simulink model "GEO_insertion"  (R2023b)
settings: Solver=FixedStepAuto  StartTime=0.0  StopTime=60*60*24*20  FixedStep=60  RelTol=1e-3
values from neighbouring files (symbols this model uses):
  A = 42164500    [GEO_insertion_setup.m]
  ext_ENV_muEarth = 3.986005e14    (= 398600500000000)    [GEO_insertion_setup.m]    (also in HSat_op_setup.m; HSat_op_setup_merged_maria.m; init_orbit_analysis_with_drag_loss.m)
  lambda_GEO = 79*pi/180    (= 1.37881010908)    [GEO_insertion_setup.m]
  OR_thrusterforce = 50e-3    (= 0.05)    [GEO_insertion_setup.m]    (also in HSat_op_setup.m = 0.275; HSat_op_setup_merged_maria.m = 0.275)
  psi_rads = 7.2921e-05    [GEO_insertion_setup.m]
  SC_mass = 500    [GEO_insertion_setup.m]
  sim_start = juliandate(2020, 1, 1, 12, 0, 0)    [GEO_insertion_setup.m]    (also in HSat_op_setup.m = ymd2jd(YYYY,MM,DD,'gregorian')-.5+hh/24+mm/1440+ss/86400; HSat_op_setup_merged_maria.m = ymd2jd(YYYY,MM,DD,'gregorian')-.5+hh/24+mm/1440+ss/86400)
  thrust_acc = OR_thrusterforce/SC_mass    (= 0.0001)    [GEO_insertion_setup.m]
undefined symbols (not defined in the file or in its folder): pos_start, vel_start
libraries: simulink x4, aerolibutil x2, sharedtransform x1, matrix_library x1
(part 1 of 2)
settings Model: Creator=mariahoflund  LastModifiedBy=mariahoflund

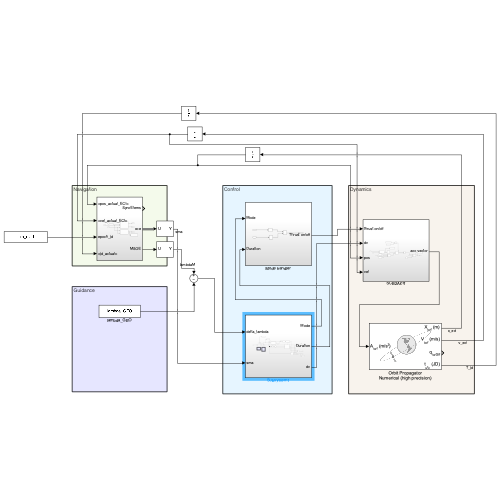
[thumbnail: Simulink's stored preview of the top-level diagram]
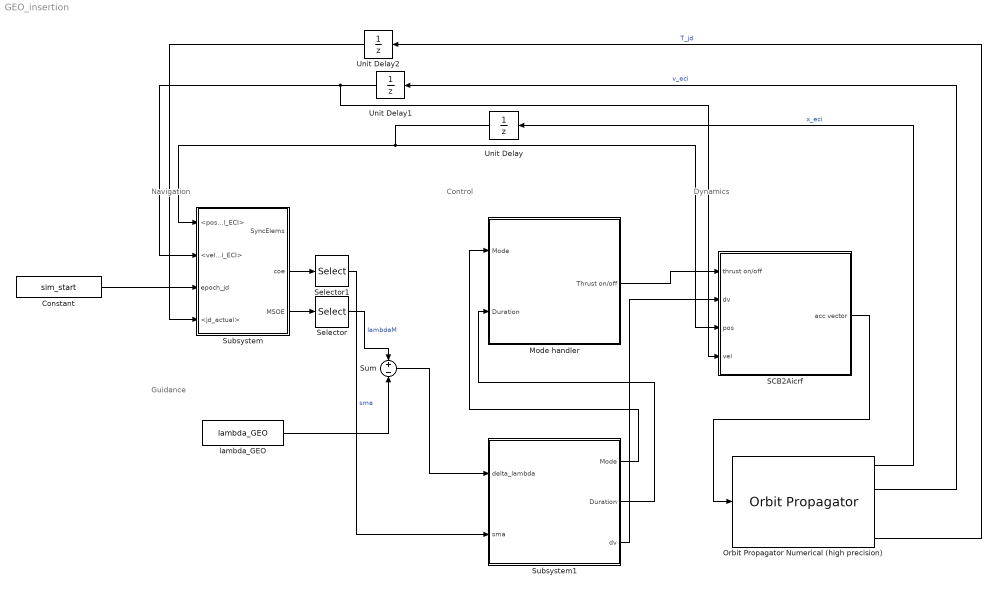
== system GEO_insertion ==
  note: Dynamics
  note: Control
  note: Navigation
  note: Guidance
  Constant : Constant  Value=sim_start
  Mode handler : Subsystem
  Orbit Propagator Numerical (high precision) : OrbitPropagator  propagator=Numerical (high precision)  accelIn=on  startDate=sim_start  semiMajorAxis=sma0  eccentricity=e0  inclination=inc0  raan=RAAN0  argPeriapsis=Arg_of_per0  trueAnomaly=nu0  inertialPosition=[3649700.0 3308200.0 -4676600.0]  inertialVelocity=[-2750.8 6666.4 2573.4]  fixedPosition=[-4142689.0 -2676864.7 -4669861.6]  fixedVelocity=[1452.7 -6720.7 2568.1]  customR=3396200  customMu=4.305e13  customJ2=1.0826269e-03  customOmega=4.06125949e-3  outputTransform=on
  SCB2Aicrf : Subsystem
  Selector : Selector  InputPortWidth=6  IndexOptions=Index vector (dialog)  Indices=[1]  OutputSizes=1
  Selector1 : Selector  InputPortWidth=11  IndexOptions=Index vector (dialog)  Indices=[1]  OutputSizes=1
  Subsystem : Subsystem
  Subsystem1 : Subsystem
  Sum : Sum  Inputs=+|-
  Unit Delay : UnitDelay  InitialCondition=pos_start  SampleTime=-1  HasFrameUpgradeWarning=on
  Unit Delay1 : UnitDelay  InitialCondition=vel_start  SampleTime=-1  HasFrameUpgradeWarning=on
  Unit Delay2 : UnitDelay  InitialCondition=sim_start  SampleTime=-1  HasFrameUpgradeWarning=on
  lambda_GEO : Constant  Value=lambda_GEO
  wires:
  Orbit Propagator Numerical (high precision)/1 -> Unit Delay/1  "x_eci"
  Orbit Propagator Numerical (high precision)/2 -> Unit Delay1/1  "v_eci"
  Orbit Propagator Numerical (high precision)/4 -> Unit Delay2/1  "T_jd"
  Unit Delay2/1 -> Subsystem/4(<jd_actual>)
  Unit Delay/1 -> Subsystem/1(<pos_actual_ECI>), SCB2Aicrf/3(pos)
  Unit Delay1/1 -> SCB2Aicrf/4(vel), Subsystem/2(<vel_actual_ECI>)
  Subsystem/3(MSOE) -> Selector/1
  Selector/1 -> Sum/1  "lambdaM"
  lambda_GEO/1 -> Sum/2
  Sum/1 -> Subsystem1/1(delta_lambda)
  Subsystem/2(coe) -> Selector1/1
  Constant/1 -> Subsystem/3(epoch_jd)
  SCB2Aicrf/1(acc vector) -> Orbit Propagator Numerical (high precision)/1
  Subsystem1/1(Mode) -> Mode handler/1(Mode)
  Subsystem1/2(Duration) -> Mode handler/2(Duration)
  Mode handler/1(Thrust on/off) -> SCB2Aicrf/1(thrust on/off)
  Subsystem1/3(dv) -> SCB2Aicrf/2(dv)
  Selector1/1 -> Subsystem1/2(sma)  "sma"

== system GEO_insertion/Mode handler ==
  Mode : Inport
  Duration : Inport  Port=2
  Compare To Constant : simulink/Logic and Bit Operations/Compare To Constant  relop===  const=2  OutDataTypeStr=boolean
  Compare To Zero : simulink/Logic and Bit Operations/Compare To Zero  relop=~=  OutDataTypeStr=boolean
  Logical Operator : Logic  AllPortsSameDT=off  OutDataTypeStr=boolean
  Thrust on/off : Outport
  wires:
  Mode/1 -> Compare To Constant/1
  Duration/1 -> Compare To Zero/1
  Compare To Constant/1 -> Logical Operator/1
  Compare To Zero/1 -> Logical Operator/2
  Logical Operator/1 -> Thrust on/off/1

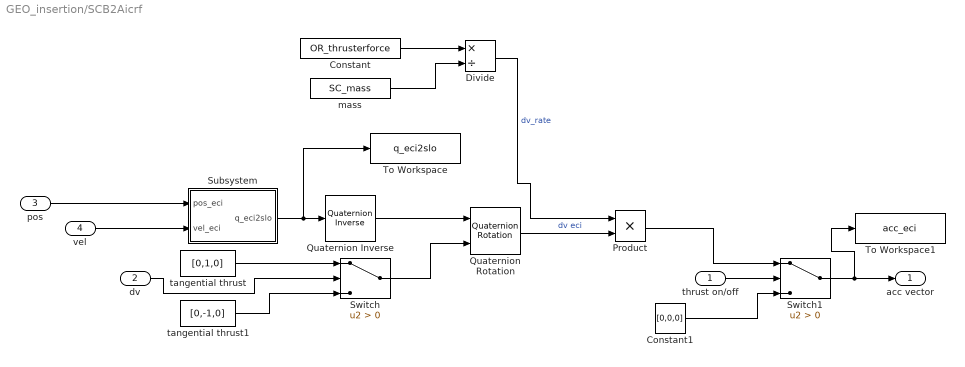
== system GEO_insertion/SCB2Aicrf ==
  thrust on/off : Inport
  dv : Inport  Port=2
  pos : Inport  Port=3
  vel : Inport  Port=4
  Constant : Constant  Value=OR_thrusterforce
  Constant1 : Constant  Value=[0,0,0]
  Divide : Product  Inputs=*/
  Product : Product
  Quaternion Inverse : aerolibutil/Quaternion Inverse
  Quaternion Rotation : aerolibutil/Quaternion Rotation
  Subsystem : Subsystem
  Switch : Switch  Criteria=u2 > Threshold  SaturateOnIntegerOverflow=off  InputSameDT=off
  Switch1 : Switch  Criteria=u2 > Threshold  SaturateOnIntegerOverflow=off  InputSameDT=off
  To Workspace : ToWorkspace  VariableName=q_eci2slo  SaveFormat=Timeseries  SampleTime=-1
  To Workspace1 : ToWorkspace  VariableName=acc_eci  SaveFormat=Timeseries  SampleTime=-1
  mass : Constant  Value=SC_mass
  tangential thrust : Constant  Value=[0,1,0]
  tangential thrust1 : Constant  Value=[0,-1,0]
  acc vector : Outport
  wires:
  pos/1 -> Subsystem/1(pos_eci)
  vel/1 -> Subsystem/2(vel_eci)
  Subsystem/1(q_eci2slo) -> To Workspace/1, Quaternion Inverse/1
  Quaternion Inverse/1 -> Quaternion Rotation/1
  Quaternion Rotation/1 -> Product/2  "dv eci"
  Constant/1 -> Divide/1
  mass/1 -> Divide/2
  Divide/1 -> Product/1  "dv_rate"
  dv/1 -> Switch/2
  tangential thrust/1 -> Switch/1
  Product/1 -> Switch1/1
  Switch/1 -> Quaternion Rotation/2
  tangential thrust1/1 -> Switch/3
  thrust on/off/1 -> Switch1/2
  Switch1/1 -> To Workspace1/1, acc vector/1
  Constant1/1 -> Switch1/3

== system GEO_insertion/Subsystem ==
  <pos_actual_ECI> : Inport
  <vel_actual_ECI> : Inport  Port=2
  epoch_jd : Inport  Port=3
  <jd_actual> : Inport  Port=4
  Subsystem : Subsystem
  Subsystem2 : Subsystem
  To Workspace : ToWorkspace  VariableName=coe  SaveFormat=Timeseries  SampleTime=-1
  SyncElems : Outport
  coe : Outport  Port=2
  MSOE : Outport  Port=3
  wires:
  <jd_actual>/1 -> Subsystem2/1(jd)
  Subsystem2/1(SyncElems) -> SyncElems/1
  epoch_jd/1 -> Subsystem2/2(epoch_jd)
  <vel_actual_ECI>/1 -> Subsystem/2(velECI), Subsystem2/4(vel_ECI)
  <pos_actual_ECI>/1 -> Subsystem/1(posECI), Subsystem2/3(pos_ECI)
  Subsystem/1(coe) -> To Workspace/1, coe/1
  Subsystem2/2(MSOE) -> MSOE/1

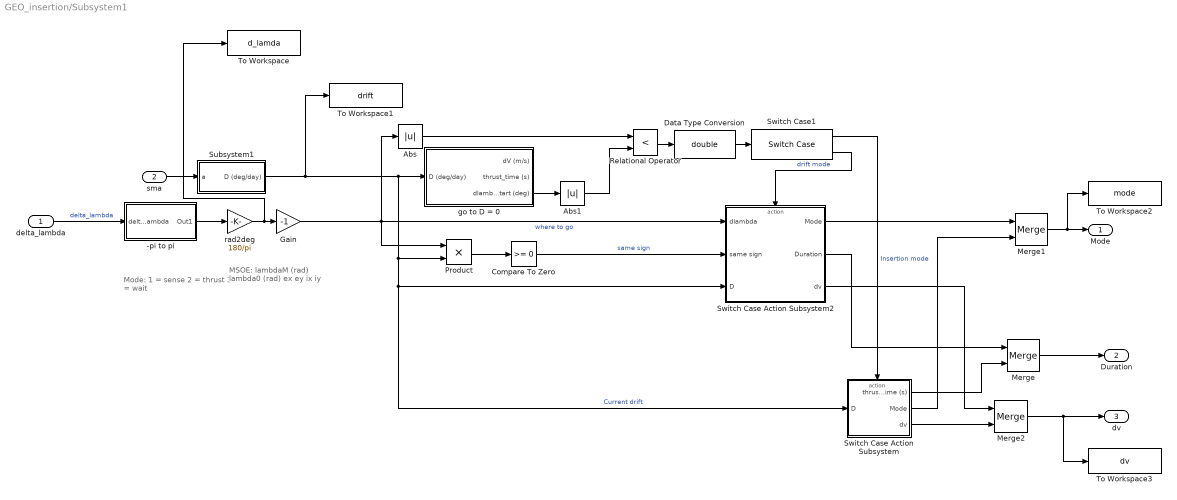
== system GEO_insertion/Subsystem1 ==
  note: Mode:
      | 1 = sense
      | 2 = thrust
      | 3 = wait
  note: MSOE:
      | lambdaM (rad)
      | lambda0 (rad)
      | ex
      | ey
      | ix
      | iy
  delta_lambda : Inport
  sma : Inport  Port=2
  -pi to pi : Subsystem
  Abs : Abs  SaturateOnIntegerOverflow=off
  Abs1 : Abs  SaturateOnIntegerOverflow=off
  Compare To Zero : simulink/Logic and Bit Operations/Compare To Zero  relop=>=  OutDataTypeStr=boolean
  Data Type Conversion : DataTypeConversion  OutDataTypeStr=double  SaturateOnIntegerOverflow=off  RndMeth=Floor
  Gain : Gain  Gain=-1
  Merge : Merge
  Merge1 : Merge
  Merge2 : Merge
  Product : Product
  Relational Operator : RelationalOperator  Operator=<  OutDataTypeStr=boolean  RndMeth=Simplest  InputSameDT=off
  Subsystem1 : Subsystem
  Switch Case Action Subsystem : Subsystem  TreatAsAtomicUnit=on
  Switch Case Action Subsystem2 : Subsystem  TreatAsAtomicUnit=on
  Switch Case1 : SwitchCase
  To Workspace : ToWorkspace  VariableName=d_lamda  SaveFormat=Timeseries  SampleTime=-1
  To Workspace1 : ToWorkspace  VariableName=drift  SaveFormat=Timeseries  SampleTime=-1
  To Workspace2 : ToWorkspace  VariableName=mode  SaveFormat=Timeseries  SampleTime=-1
  To Workspace3 : ToWorkspace  VariableName=dv  SaveFormat=Timeseries  SampleTime=-1
  go to D = 0 : Subsystem
  rad2deg : Gain  Gain=180/pi
  Mode : Outport
  Duration : Outport  Port=2
  dv : Outport  Port=3
  wires:
  delta_lambda/1 -> -pi to pi/1(delta_lambda)  "delta_lambda"
  -pi to pi/1(Out1) -> rad2deg/1
  rad2deg/1 -> To Workspace/1, Gain/1
  Gain/1 -> Product/1, Switch Case Action Subsystem2/1(dlambda), Abs/1  "where to go"
  Product/1 -> Compare To Zero/1
  Compare To Zero/1 -> Switch Case Action Subsystem2/2(same sign)  "same sign"
  Subsystem1/1(D (deg/day)) -> To Workspace1/1, go to D = 0/1(D (deg/day)), Product/2, Switch Case Action Subsystem2/3(D), Switch Case Action Subsystem/1(D)  "Current drift"
  sma/1 -> Subsystem1/1(a)
  go to D = 0/3(dlambda_start (deg)) -> Abs1/1
  Relational Operator/1 -> Data Type Conversion/1
  Switch Case1/2 -> Switch Case Action Subsystem2/Action  "drift mode"
  Switch Case1/1 -> Switch Case Action Subsystem/Action  "Insertion mode"
  Switch Case Action Subsystem/1(thrust_time (s)) -> Merge/2
  Switch Case Action Subsystem2/2(Duration) -> Merge/1
  Merge/1 -> Duration/1
  Switch Case Action Subsystem/2(Mode) -> Merge1/2
  Switch Case Action Subsystem2/1(Mode) -> Merge1/1
  Merge1/1 -> To Workspace2/1, Mode/1
  Switch Case Action Subsystem2/3(dv) -> Merge2/1
  Switch Case Action Subsystem/3(dv) -> Merge2/2
  Merge2/1 -> To Workspace3/1, dv/1
  Data Type Conversion/1 -> Switch Case1/1
  Abs/1 -> Relational Operator/1
  Abs1/1 -> Relational Operator/2

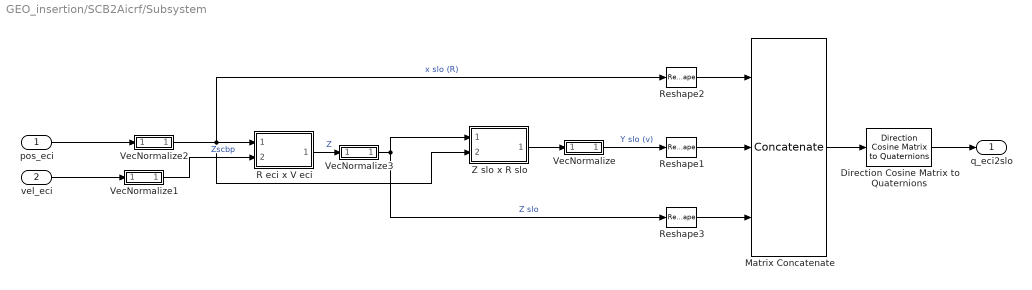
== system GEO_insertion/SCB2Aicrf/Subsystem ==
  pos_eci : Inport
  vel_eci : Inport  Port=2
  Direction Cosine Matrix to Quaternions : sharedtransform/Direction Cosine Matrix  to Quaternions  aMode=0  action=None  tolerance=eps(2)
      settings: LibrarySourceBlock=|
      | aerolibtransform2/Direction Cosine Matrix
      | to Quaternions
  Matrix Concatenate : Concatenate  NumInputs=3  Mode=Multidimensional array
  R eci x V eci : Subsystem  mask(Cross Product){}
      mask help: Calculates the cross product of two 3x1 vectors.
      mask Help:
      | <p>This block calculates the cross product of two 3x1 vectors, ie.</p>
      | 
      | <ul>C(1) = A(2)*B(3) - A(3)*B(2)</ul>
      | <ul>C(2) = A(3)*B(1) - A(1)*B(3)</ul>
      | <ul>C(3) = A(1)*B(2) - A(2)*B(1)</ul>
      | 
      | <p>The block inputs and output contain more than one signal as described below.</p>
      | 
      | <p><H4>Block Vector Input 1 - A</H4>
      | <ul>
      | <li>A(1)</li>
      | <li>A(2)</li>
      | <li>A(3)</li>
      | </ul>
      | </p>
      | 
      | <p><H4>Block Vector Input 2 - B</H4>
      | <ul>
      | <li>B(1)</li>
      | <li>B(2)</li>
      | <li>B(3)</li>
      | </ul>
      | </p>
      | 
      | <p><H4>Block Vector Output - Cross Product (AxB)</H4>
      | <ul>
      | <li>C(1)</li>
      | <li>C(2)</li>
      | <li>C(3)</li>
      | </ul>
      | </p>
      mask Display: disp('Cross\nProduct')
  Reshape1 : Reshape  OutputDimensionality=Row vector (2-D)
  Reshape2 : Reshape  OutputDimensionality=Row vector (2-D)
  Reshape3 : Reshape  OutputDimensionality=Row vector (2-D)
  VecNormalize : Subsystem
      mask Display: disp('u/||u||')
  VecNormalize1 : Subsystem
      mask Display: disp('u/||u||')
  VecNormalize2 : Subsystem
      mask Display: disp('u/||u||')
  VecNormalize3 : Subsystem
      mask Display: disp('u/||u||')
  Z slo x R slo : Subsystem  mask(Cross Product){}
      mask help: Calculates the cross product of two 3x1 vectors.
      mask Help:
      | <p>This block calculates the cross product of two 3x1 vectors, ie.</p>
      | 
      | <ul>C(1) = A(2)*B(3) - A(3)*B(2)</ul>
      | <ul>C(2) = A(3)*B(1) - A(1)*B(3)</ul>
      | <ul>C(3) = A(1)*B(2) - A(2)*B(1)</ul>
      | 
      | <p>The block inputs and output contain more than one signal as described below.</p>
      | 
      | <p><H4>Block Vector Input 1 - A</H4>
      | <ul>
      | <li>A(1)</li>
      | <li>A(2)</li>
      | <li>A(3)</li>
      | </ul>
      | </p>
      | 
      | <p><H4>Block Vector Input 2 - B</H4>
      | <ul>
      | <li>B(1)</li>
      | <li>B(2)</li>
      | <li>B(3)</li>
      | </ul>
      | </p>
      | 
      | <p><H4>Block Vector Output - Cross Product (AxB)</H4>
      | <ul>
      | <li>C(1)</li>
      | <li>C(2)</li>
      | <li>C(3)</li>
      | </ul>
      | </p>
      mask Display: disp('Cross\nProduct')
  q_eci2slo : Outport
  wires:
  pos_eci/1 -> VecNormalize2/1(In1)
  vel_eci/1 -> VecNormalize1/1(In1)
  Reshape2/1 -> Matrix Concatenate/1
  VecNormalize/1(Out1) -> Reshape1/1  "Y slo (v)"
  Reshape3/1 -> Matrix Concatenate/3
  VecNormalize1/1(Out1) -> R eci x V eci/2(b(1) b(2) b(3))  "Zscbp"
  R eci x V eci/1(c(1) c(2) c(3)) -> VecNormalize3/1(In1)  "Z"
  Z slo x R slo/1(c(1) c(2) c(3)) -> VecNormalize/1(In1)
  Matrix Concatenate/1 -> Direction Cosine Matrix to Quaternions/1
  Reshape1/1 -> Matrix Concatenate/2
  Direction Cosine Matrix to Quaternions/1 -> q_eci2slo/1
  VecNormalize3/1(Out1) -> Z slo x R slo/1(a(1) a(2) a(3)), Reshape3/1  "Z slo"
  VecNormalize2/1(Out1) -> Reshape2/1, Z slo x R slo/2(b(1) b(2) b(3)), R eci x V eci/1(a(1) a(2) a(3))  "x slo (R)"

== system GEO_insertion/Subsystem/Subsystem ==
  posECI : Inport
  velECI : Inport  Port=2
  Bus Creator : BusCreator  Inputs=11
  Demux : Demux  Outputs=11
  MATLAB Function : MATLAB Function  TreatAsAtomicUnit=on
  coe : Outport
  wires:
  posECI/1 -> MATLAB Function/1(r)
  Demux/10 -> Bus Creator/10  "truelong"
  Demux/1 -> Bus Creator/1  "sms"
  Demux/3 -> Bus Creator/3  "incl"
  Demux/7 -> Bus Creator/7  "eccan"
  Demux/9 -> Bus Creator/9  "arglat"
  Demux/4 -> Bus Creator/4  "raan"
  Demux/2 -> Bus Creator/2  "ecc"
  Demux/11 -> Bus Creator/11  "longper"
  Demux/6 -> Bus Creator/6  "truean"
  MATLAB Function/1(coe) -> Demux/1
  Bus Creator/1 -> coe/1  "coe"
  velECI/1 -> MATLAB Function/2(v)
  Demux/5 -> Bus Creator/5  "argp"
  Demux/8 -> Bus Creator/8  "meanan"

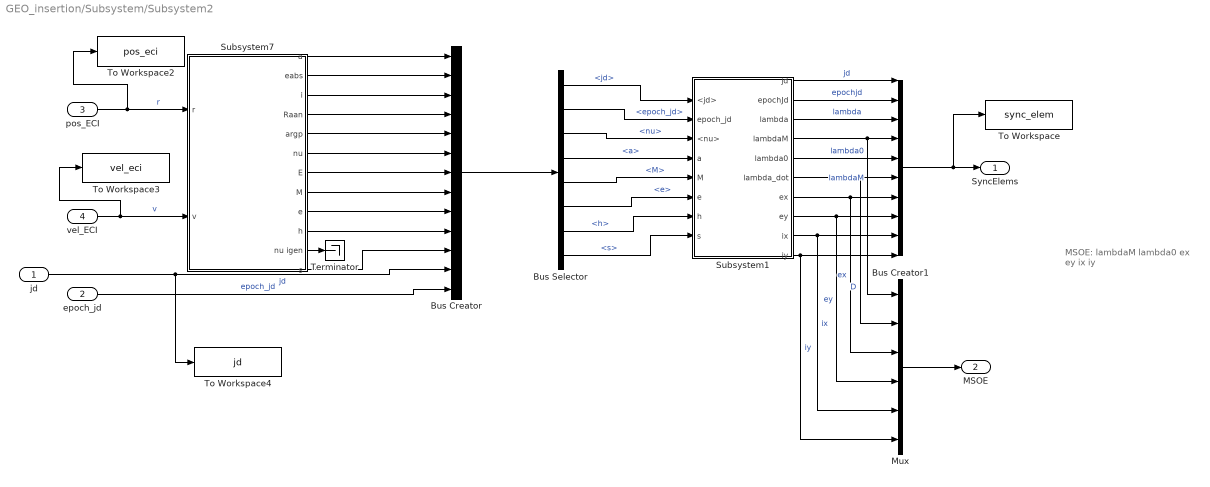
== system GEO_insertion/Subsystem/Subsystem2 ==
  note: MSOE:
      | lambdaM
      | lambda0
      | ex
      | ey
      | ix
      | iy
  jd : Inport
  epoch_jd : Inport  Port=2
  pos_ECI : Inport  Port=3
  vel_ECI : Inport  Port=4
  Bus Creator : BusCreator  Inputs=13
  Bus Creator1 : BusCreator  Inputs=10
  Bus Selector : BusSelector  OutputSignals=jd,epoch_jd,nu,a,M,e,h,s
  Mux : Mux  Inputs=6
  Subsystem1 : Subsystem
  Subsystem7 : Subsystem
  Terminator : Terminator
  To Workspace : ToWorkspace  VariableName=sync_elem  SaveFormat=Timeseries  SampleTime=-1
  To Workspace2 : ToWorkspace  VariableName=pos_eci  SaveFormat=Timeseries  SampleTime=-1
  To Workspace3 : ToWorkspace  VariableName=vel_eci  SaveFormat=Timeseries  SampleTime=-1
  To Workspace4 : ToWorkspace  VariableName=jd  SaveFormat=Timeseries  SampleTime=-1
  SyncElems : Outport
  MSOE : Outport  Port=2
  wires:
  pos_ECI/1 -> To Workspace2/1, Subsystem7/1(r)  "r"
  vel_ECI/1 -> To Workspace3/1, Subsystem7/2(v)  "v"
  Subsystem7/9(e) -> Bus Creator/9
  Subsystem7/2(eabs) -> Bus Creator/2
  Subsystem7/10(h) -> Bus Creator/10
  Subsystem7/3(i) -> Bus Creator/3
  Subsystem7/5(argp) -> Bus Creator/5
  Subsystem7/4(Raan) -> Bus Creator/4
  Subsystem7/1(a) -> Bus Creator/1
  Subsystem7/6(nu) -> Bus Creator/6
  jd/1 -> To Workspace4/1, Bus Creator/12  "jd"
  Bus Creator/1 -> Bus Selector/1
  Bus Selector/1 -> Subsystem1/1(<jd>)  "<jd>"
  Bus Selector/3 -> Subsystem1/3(<nu>)  "<nu>"
  Subsystem7/8(M) -> Bus Creator/8
  Subsystem7/7(E) -> Bus Creator/7
  Subsystem7/11(nu igen) -> Terminator/1
  epoch_jd/1 -> Bus Creator/13  "epoch_jd"
  Bus Selector/2 -> Subsystem1/2(epoch_jd)  "<epoch_jd>"
  Bus Selector/5 -> Subsystem1/5(M)  "<M>"
  Bus Selector/4 -> Subsystem1/4(a)  "<a>"
  Bus Selector/6 -> Subsystem1/6(e)  "<e>"
  Bus Selector/7 -> Subsystem1/7(h)  "<h>"
  Subsystem1/1(jd) -> Bus Creator1/1  "jd"
  Subsystem1/2(epochJd) -> Bus Creator1/2  "epochjd"
  Subsystem1/3(lambda) -> Bus Creator1/3  "lambda"
  Subsystem1/4(lambdaM) -> Mux/1, Bus Creator1/4  "lambdaM"
  Subsystem1/5(lambda0) -> Bus Creator1/5  "lambda0"
  Subsystem1/6(lambda_dot) -> Mux/2, Bus Creator1/6  "D"
  Subsystem1/7(ex) -> Mux/3, Bus Creator1/7  "ex"
  Subsystem1/9(ix) -> Mux/5, Bus Creator1/9  "ix"
  Bus Creator1/1 -> To Workspace/1, SyncElems/1
  Subsystem1/8(ey) -> Mux/4, Bus Creator1/8  "ey"
  Subsystem1/10(iy) -> Mux/6, Bus Creator1/10  "iy"
  Subsystem7/12(s) -> Bus Creator/11
  Bus Selector/8 -> Subsystem1/8(s)  "<s>"
  Mux/1 -> MSOE/1

== system GEO_insertion/Subsystem1/-pi to pi ==
  delta_lambda : Inport
  Add : Sum
  Add1 : Sum
  Constant : Constant  Value=pi
  Constant1 : Constant  Value=2*pi
  Constant2 : Constant  Value=pi
  Constant3 : Constant  Value=2*pi
  Subtract : Sum  Inputs=+-
  Subtract1 : Sum  Inputs=+-
  Switch : Switch  Criteria=u2 > Threshold  SaturateOnIntegerOverflow=off  InputSameDT=off
  Switch1 : Switch  Criteria=u2 > Threshold  SaturateOnIntegerOverflow=off  InputSameDT=off
  Switch2 : Switch  Criteria=u2 > Threshold  SaturateOnIntegerOverflow=off  InputSameDT=off
  Out1 : Outport
  wires:
  delta_lambda/1 -> Add1/1, Switch1/1, Add/1, Switch2/2, Switch/3, Subtract1/1, Subtract/1
  Constant/1 -> Subtract/2
  Subtract/1 -> Switch/2
  Constant1/1 -> Subtract1/2
  Subtract1/1 -> Switch/1
  Switch/1 -> Switch2/1
  Constant2/1 -> Add/2
  Add/1 -> Switch1/2
  Constant3/1 -> Add1/2
  Add1/1 -> Switch1/3
  Switch1/1 -> Switch2/3
  Switch2/1 -> Out1/1

== system GEO_insertion/Subsystem1/Subsystem1 ==
  a : Inport
  A : Constant  Value=A
  Constant2 : Constant  Value=-1.5*361
  Divide2 : Product  Inputs=**/
  Subtract : Sum  Inputs=+-
  D (deg/day) : Outport
  wires:
  Divide2/1 -> D (deg/day)/1  "current drift"
  Constant2/1 -> Divide2/2
  Subtract/1 -> Divide2/1  "delta_a0"
  a/1 -> Subtract/1
  A/1 -> Divide2/3, Subtract/2

== system GEO_insertion/Subsystem1/Switch Case Action Subsystem ==
  D : Inport
  Action Port : ActionPort  ActionPortLabel=case [ 1 ]:
  Thrust : Constant  Value=2
  go to D = 0 : Subsystem
  thrust_time (s) : Outport
  Mode : Outport  Port=2
  dv : Outport  Port=3
  wires:
  D/1 -> go to D = 0/1(D)
  go to D = 0/2(thrust_time (s)) -> thrust_time (s)/1
  Thrust/1 -> Mode/1
  go to D = 0/1(dV (m/s)) -> dv/1

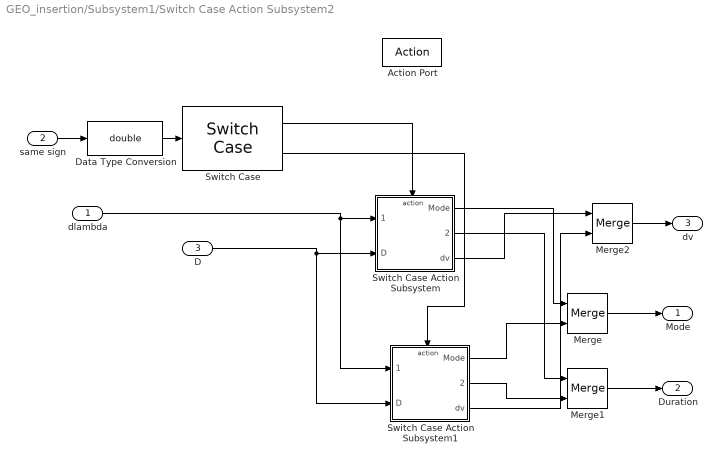
== system GEO_insertion/Subsystem1/Switch Case Action Subsystem2 ==
  dlambda : Inport
  same sign : Inport  Port=2
  D : Inport  Port=3
  Action Port : ActionPort  ActionPortLabel=default:
  Data Type Conversion : DataTypeConversion  OutDataTypeStr=double  SaturateOnIntegerOverflow=off  RndMeth=Floor
  Merge : Merge
  Merge1 : Merge
  Merge2 : Merge
  Switch Case : SwitchCase  CaseConditions={1, 0}  ShowDefaultCase=off
  Switch Case Action Subsystem : Subsystem  TreatAsAtomicUnit=on
  Switch Case Action Subsystem1 : Subsystem  TreatAsAtomicUnit=on
  Mode : Outport
  Duration : Outport  Port=2
  dv : Outport  Port=3
  wires:
  Merge1/1 -> Duration/1
  Switch Case/2 -> Switch Case Action Subsystem1/Action
  Merge/1 -> Mode/1
  Switch Case Action Subsystem1/2(duration (s)) -> Merge1/2
  D/1 -> Switch Case Action Subsystem1/2(D), Switch Case Action Subsystem/2(D)
  Switch Case Action Subsystem/2(duration (s)) -> Merge1/1
  Switch Case/1 -> Switch Case Action Subsystem/Action
  dlambda/1 -> Switch Case Action Subsystem1/1(dlambda), Switch Case Action Subsystem/1(dlambda)
  Switch Case Action Subsystem/1(Mode) -> Merge/1
  Switch Case Action Subsystem1/1(Mode) -> Merge/2
  same sign/1 -> Data Type Conversion/1
  Switch Case Action Subsystem/3(dv) -> Merge2/1
  Switch Case Action Subsystem1/3(dv) -> Merge2/2
  Merge2/1 -> dv/1
  Data Type Conversion/1 -> Switch Case/1

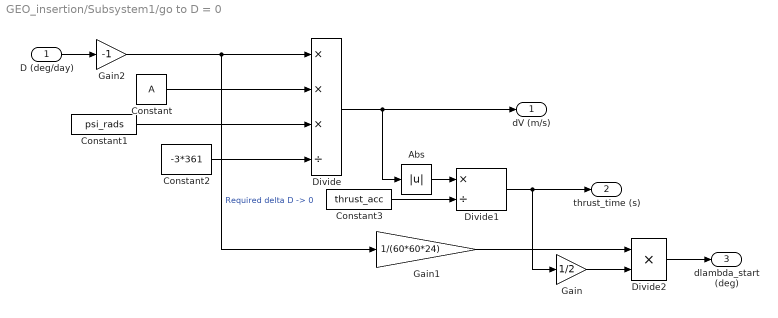
== system GEO_insertion/Subsystem1/go to D = 0 ==
  D (deg/day) : Inport
  Abs : Abs  SaturateOnIntegerOverflow=off
  Constant : Constant  Value=A
  Constant1 : Constant  Value=psi_rads
  Constant2 : Constant  Value=-3*361
  Constant3 : Constant  Value=thrust_acc
  Divide : Product  Inputs=***/
  Divide1 : Product  Inputs=*/
  Divide2 : Product  Inputs=**
  Gain : Gain  Gain=1/2
  Gain1 : Gain  Gain=1/(60*60*24)
  Gain2 : Gain  Gain=-1
  dV (m/s) : Outport
  thrust_time (s) : Outport  Port=2
  dlambda_start (deg) : Outport  Port=3
  wires:
  D (deg/day)/1 -> Gain2/1
  Constant/1 -> Divide/2
  Constant1/1 -> Divide/3
  Constant2/1 -> Divide/4
  Divide/1 -> dV (m/s)/1, Abs/1
  Constant3/1 -> Divide1/2
  Divide1/1 -> Gain/1, thrust_time (s)/1
  Gain/1 -> Divide2/2
  Divide2/1 -> dlambda_start (deg)/1
  Gain1/1 -> Divide2/1
  Gain2/1 -> Gain1/1, Divide/1  "Required delta D -> 0"
  Abs/1 -> Divide1/1

== system GEO_insertion/SCB2Aicrf/Subsystem/R eci x V eci ==
  a(1) a(2) a(3) : Inport
  b(1) b(2) b(3) : Inport  Port=2
  Product : Product  InputSameDT=on  SaturateOnIntegerOverflow=on  OutDataTypeStr=Inherit: Same as first input
  Product1 : Product  InputSameDT=on  SaturateOnIntegerOverflow=on  OutDataTypeStr=Inherit: Same as first input
  Selector : Selector  InputPortWidth=3  IndexOptions=Index vector (dialog)  Indices=[2 3 1]  OutputSizes=1
  Selector1 : Selector  InputPortWidth=3  IndexOptions=Index vector (dialog)  Indices=[3 1 2]  OutputSizes=1
  Selector2 : Selector  InputPortWidth=3  IndexOptions=Index vector (dialog)  Indices=[2 3 1]  OutputSizes=1
  Selector3 : Selector  InputPortWidth=3  IndexOptions=Index vector (dialog)  Indices=[3 1 2]  OutputSizes=1
  Sum : Sum  Inputs=+|-  InputSameDT=on  SaturateOnIntegerOverflow=on  OutDataTypeStr=Inherit: Same as first input
  c(1) c(2) c(3) : Outport  InitialOutput=0
  wires:
  Selector3/1 -> Product1/1
  Selector2/1 -> Product1/2
  Product1/1 -> Sum/2
  Selector1/1 -> Product/2
  Product/1 -> Sum/1
  a(1) a(2) a(3)/1 -> Selector3/1, Selector/1
  Selector/1 -> Product/1
  b(1) b(2) b(3)/1 -> Selector2/1, Selector1/1
  Sum/1 -> c(1) c(2) c(3)/1

== system GEO_insertion/SCB2Aicrf/Subsystem/VecNormalize ==
  In1 : Inport
  Constant : Constant
  Demux : Demux  Outputs=[-1 1]
  Divide : Product  Inputs=*/  OutDataTypeStr=double
  Ground : Ground
  Math Function : Math  Operator=square  SignedPower=on
  Math Function1 : Math  Operator=sqrt  SignedPower=on
  Mux : Mux  Inputs=2
  Mux1 : Mux  Inputs=2
  Product : Product  RndMeth=Zero
  Sum of Elements : Sum  Inputs=+
  Switch : Switch  Criteria=u2 > Threshold  Threshold=eps  SaturateOnIntegerOverflow=off  InputSameDT=off
  Out1 : Outport  VectorParamsAs1DForOutWhenUnconnected=off
  wires:
  Math Function/1 -> Sum of Elements/1
  Demux/1 -> Divide/1
  Constant/1 -> Mux1/2
  Mux1/1 -> Switch/3
  Divide/1 -> Out1/1
  Switch/1 -> Demux/1
  Mux/1 -> Switch/1
  Demux/2 -> Divide/2
  Product/1 -> Mux1/1
  In1/1 -> Product/1, Math Function/1, Mux/1
  Ground/1 -> Product/2
  Sum of Elements/1 -> Math Function1/1
  Math Function1/1 -> Mux/2, Switch/2

== system GEO_insertion/SCB2Aicrf/Subsystem/VecNormalize1 ==
  In1 : Inport
  Constant : Constant
  Demux : Demux  Outputs=[-1 1]
  Divide : Product  Inputs=*/  OutDataTypeStr=double
  Ground : Ground
  Math Function : Math  Operator=square  SignedPower=on
  Math Function1 : Math  Operator=sqrt  SignedPower=on
  Mux : Mux  Inputs=2
  Mux1 : Mux  Inputs=2
  Product : Product  RndMeth=Zero
  Sum of Elements : Sum  Inputs=+
  Switch : Switch  Criteria=u2 > Threshold  Threshold=eps  SaturateOnIntegerOverflow=off  InputSameDT=off
  Out1 : Outport  VectorParamsAs1DForOutWhenUnconnected=off
  wires:
  Math Function/1 -> Sum of Elements/1
  Demux/1 -> Divide/1
  Constant/1 -> Mux1/2
  Mux1/1 -> Switch/3
  Divide/1 -> Out1/1
  Switch/1 -> Demux/1
  Mux/1 -> Switch/1
  Demux/2 -> Divide/2
  Product/1 -> Mux1/1
  In1/1 -> Product/1, Math Function/1, Mux/1
  Ground/1 -> Product/2
  Sum of Elements/1 -> Math Function1/1
  Math Function1/1 -> Mux/2, Switch/2

== system GEO_insertion/SCB2Aicrf/Subsystem/VecNormalize2 ==
  In1 : Inport
  Constant : Constant
  Demux : Demux  Outputs=[-1 1]
  Divide : Product  Inputs=*/  OutDataTypeStr=double
  Ground : Ground
  Math Function : Math  Operator=square  SignedPower=on
  Math Function1 : Math  Operator=sqrt  SignedPower=on
  Mux : Mux  Inputs=2
  Mux1 : Mux  Inputs=2
  Product : Product  RndMeth=Zero
  Sum of Elements : Sum  Inputs=+
  Switch : Switch  Criteria=u2 > Threshold  Threshold=eps  SaturateOnIntegerOverflow=off  InputSameDT=off
  Out1 : Outport  VectorParamsAs1DForOutWhenUnconnected=off
  wires:
  Math Function/1 -> Sum of Elements/1
  Demux/1 -> Divide/1
  Constant/1 -> Mux1/2
  Mux1/1 -> Switch/3
  Divide/1 -> Out1/1
  Switch/1 -> Demux/1
  Mux/1 -> Switch/1
  Demux/2 -> Divide/2
  Product/1 -> Mux1/1
  In1/1 -> Product/1, Math Function/1, Mux/1
  Ground/1 -> Product/2
  Sum of Elements/1 -> Math Function1/1
  Math Function1/1 -> Mux/2, Switch/2

== system GEO_insertion/SCB2Aicrf/Subsystem/VecNormalize3 ==
  In1 : Inport
  Constant : Constant
  Demux : Demux  Outputs=[-1 1]
  Divide : Product  Inputs=*/  OutDataTypeStr=double
  Ground : Ground
  Math Function : Math  Operator=square  SignedPower=on
  Math Function1 : Math  Operator=sqrt  SignedPower=on
  Mux : Mux  Inputs=2
  Mux1 : Mux  Inputs=2
  Product : Product  RndMeth=Zero
  Sum of Elements : Sum  Inputs=+
  Switch : Switch  Criteria=u2 > Threshold  Threshold=eps  SaturateOnIntegerOverflow=off  InputSameDT=off
  Out1 : Outport  VectorParamsAs1DForOutWhenUnconnected=off
  wires:
  Math Function/1 -> Sum of Elements/1
  Demux/1 -> Divide/1
  Constant/1 -> Mux1/2
  Mux1/1 -> Switch/3
  Divide/1 -> Out1/1
  Switch/1 -> Demux/1
  Mux/1 -> Switch/1
  Demux/2 -> Divide/2
  Product/1 -> Mux1/1
  In1/1 -> Product/1, Math Function/1, Mux/1
  Ground/1 -> Product/2
  Sum of Elements/1 -> Math Function1/1
  Math Function1/1 -> Mux/2, Switch/2

== system GEO_insertion/SCB2Aicrf/Subsystem/Z slo x R slo ==
  a(1) a(2) a(3) : Inport
  b(1) b(2) b(3) : Inport  Port=2
  Product : Product  InputSameDT=on  SaturateOnIntegerOverflow=on  OutDataTypeStr=Inherit: Same as first input
  Product1 : Product  InputSameDT=on  SaturateOnIntegerOverflow=on  OutDataTypeStr=Inherit: Same as first input
  Selector : Selector  InputPortWidth=3  IndexOptions=Index vector (dialog)  Indices=[2 3 1]  OutputSizes=1
  Selector1 : Selector  InputPortWidth=3  IndexOptions=Index vector (dialog)  Indices=[3 1 2]  OutputSizes=1
  Selector2 : Selector  InputPortWidth=3  IndexOptions=Index vector (dialog)  Indices=[2 3 1]  OutputSizes=1
  Selector3 : Selector  InputPortWidth=3  IndexOptions=Index vector (dialog)  Indices=[3 1 2]  OutputSizes=1
  Sum : Sum  Inputs=+|-  InputSameDT=on  SaturateOnIntegerOverflow=on  OutDataTypeStr=Inherit: Same as first input
  c(1) c(2) c(3) : Outport  InitialOutput=0
  wires:
  Sum/1 -> c(1) c(2) c(3)/1
  b(1) b(2) b(3)/1 -> Selector1/1, Selector2/1
  Selector/1 -> Product/1
  a(1) a(2) a(3)/1 -> Selector/1, Selector3/1
  Product/1 -> Sum/1
  Selector1/1 -> Product/2
  Product1/1 -> Sum/2
  Selector2/1 -> Product1/2
  Selector3/1 -> Product1/1

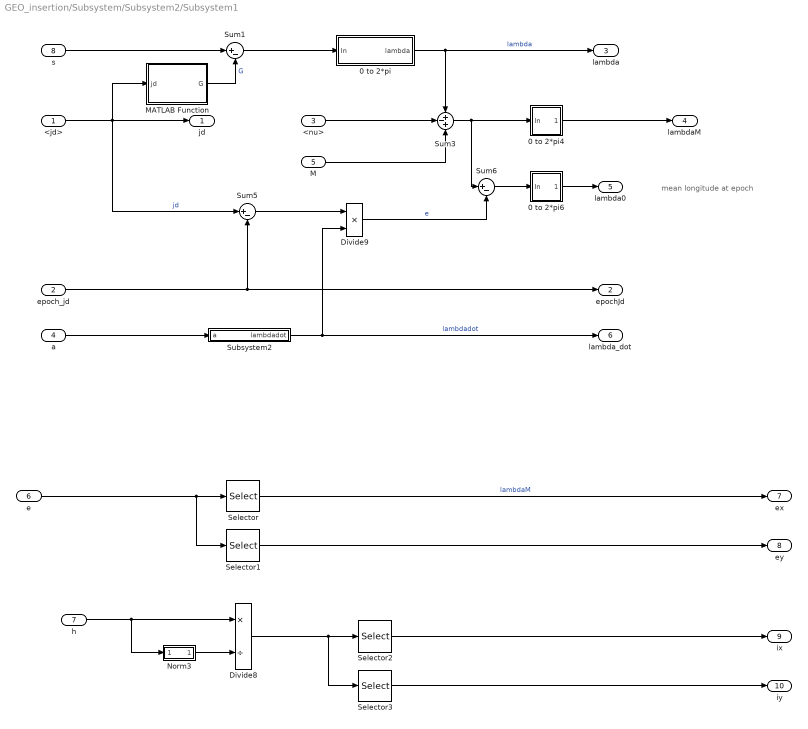
== system GEO_insertion/Subsystem/Subsystem2/Subsystem1 ==
  note: mean longitude at epoch
  <jd> : Inport
  epoch_jd : Inport  Port=2
  <nu> : Inport  Port=3
  a : Inport  Port=4
  M : Inport  Port=5
  e : Inport  Port=6
  h : Inport  Port=7
  s : Inport  Port=8
  0 to 2*pi : Subsystem
  0 to 2*pi4 : Subsystem
  0 to 2*pi6 : Subsystem
  Divide8 : Product  Inputs=*/
  Divide9 : Product  Inputs=**
  MATLAB Function : MATLAB Function  TreatAsAtomicUnit=on
  Norm3 : Subsystem  Tag=||u||
      mask Display: disp('||u||')
  Selector : Selector  InputPortWidth=3  IndexOptions=Index vector (dialog)  Indices=[1]  OutputSizes=1
  Selector1 : Selector  InputPortWidth=3  IndexOptions=Index vector (dialog)  Indices=[2]  OutputSizes=1
  Selector2 : Selector  InputPortWidth=3  IndexOptions=Index vector (dialog)  Indices=[1]  OutputSizes=1
  Selector3 : Selector  InputPortWidth=3  IndexOptions=Index vector (dialog)  Indices=[2]  OutputSizes=1
  Subsystem2 : Subsystem
  Sum1 : Sum  Inputs=|+-
  Sum3 : Sum  Inputs=+-+
  Sum5 : Sum  Inputs=|+-
  Sum6 : Sum  Inputs=|+-
  jd : Outport
  epochJd : Outport  Port=2
  lambda : Outport  Port=3
  lambdaM : Outport  Port=4
  lambda0 : Outport  Port=5
  lambda_dot : Outport  Port=6
  ex : Outport  Port=7
  ey : Outport  Port=8
  ix : Outport  Port=9
  iy : Outport  Port=10
  wires:
  <nu>/1 -> Sum3/2
  a/1 -> Subsystem2/1(a)
  M/1 -> Sum3/3
  epoch_jd/1 -> epochJd/1, Sum5/2
  Sum5/1 -> Divide9/1
  Subsystem2/1(lambdadot) -> lambda_dot/1, Divide9/2  "lambdadot"
  Divide9/1 -> Sum6/2  "e"
  e/1 -> Selector1/1, Selector/1
  Selector1/1 -> ey/1
  Selector/1 -> ex/1  "lambdaM"
  Divide8/1 -> Selector3/1, Selector2/1
  Selector3/1 -> iy/1
  Selector2/1 -> ix/1
  Norm3/1(Out1) -> Divide8/2
  h/1 -> Norm3/1(In1), Divide8/1
  Sum3/1 -> Sum6/1, 0 to 2*pi4/1(In)
  Sum6/1 -> 0 to 2*pi6/1(In)
  0 to 2*pi6/1(Out) -> lambda0/1
  <jd>/1 -> jd/1, Sum5/1, MATLAB Function/1(jd)  "jd"
  MATLAB Function/1(G) -> Sum1/2  "G"
  s/1 -> Sum1/1
  Sum1/1 -> 0 to 2*pi/1(In)
  0 to 2*pi/1(lambda) -> Sum3/1, lambda/1  "lambda"
  0 to 2*pi4/1(Out) -> lambdaM/1

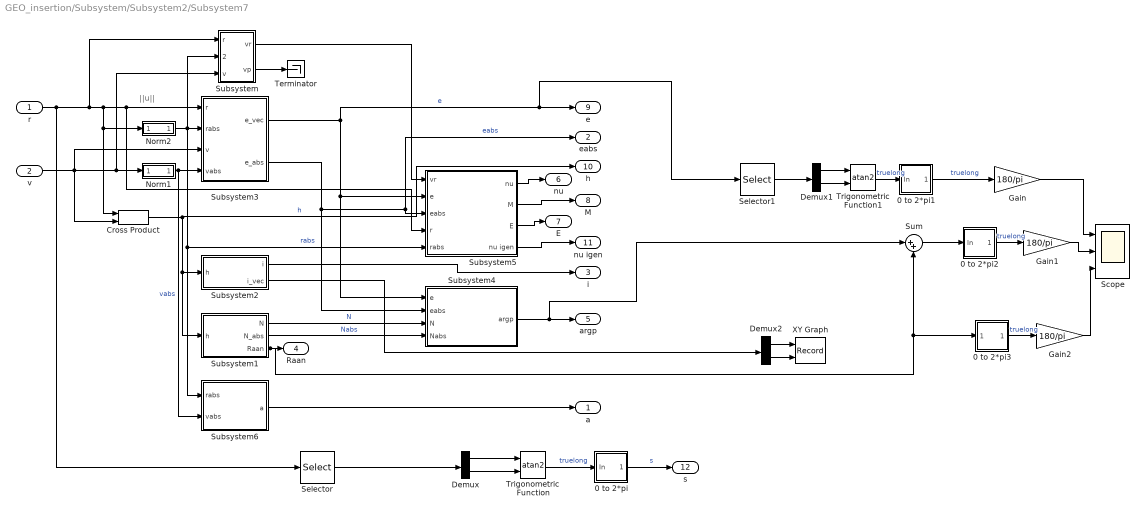
== system GEO_insertion/Subsystem/Subsystem2/Subsystem7 ==
  note: ||u||
  r : Inport
  v : Inport  Port=2
  0 to 2*pi : Subsystem
  0 to 2*pi1 : Subsystem
  0 to 2*pi2 : Subsystem
  0 to 2*pi3 : Subsystem
  Cross Product : matrix_library/Cross Product
  Demux : Demux  Outputs=2
  Demux1 : Demux  Outputs=2
  Demux2 : Demux  Outputs=2
  Gain : Gain  Gain=180/pi
  Gain1 : Gain  Gain=180/pi
  Gain2 : Gain  Gain=180/pi
  Norm1 : Subsystem  Tag=||u||
      mask Display: disp('||u||')
  Norm2 : Subsystem  Tag=||u||
      mask Display: disp('||u||')
  Scope : Scope  NumInputPorts=3
  Selector : Selector  InputPortWidth=3  IndexOptions=Index vector (dialog)  Indices=[2 1]  OutputSizes=1
  Selector1 : Selector  InputPortWidth=3  IndexOptions=Index vector (dialog)  Indices=[2 1]  OutputSizes=1
  Subsystem : Subsystem
  Subsystem1 : Subsystem
  Subsystem2 : Subsystem
  Subsystem3 : Subsystem
  Subsystem4 : Subsystem
  Subsystem5 : Subsystem
  Subsystem6 : Subsystem
  Sum : Sum  Inputs=|++
  Terminator : Terminator
  Trigonometric Function : Trigonometry  Operator=atan2
  Trigonometric Function1 : Trigonometry  Operator=atan2
  XY Graph : Record  FileSettingsInternal="{\"entries\":[{\"content\":{\"excelSettings\":{\"content\":{},\"type\":\"Streamout.ExcelSettings\"}},\"type\":\"Streamout.FileSettingStorage\",\"uuid\":\"\"}],\"packageUris\":[\"http:\\/\\/schema.mathworks.com\\/mf0\\/streamout_blocks\\/R2020a\"],\"version\":\"1.0\"}"  Layout=[1 1]  SignalsInternal="{\"entries\":[{\"content\":{\"signals\":[{\"content\":{\"blockPath\":[],\"dimensions\":[1],\"domain\":\"\",\"lineColor\":\"#a2142f\",\"plots\":[1],\"port\":1,\"sid\":[\"\"],\"signalID\":1087,\"signalName\":\"Demux2:1\"},\"type\":\"RecordBlkView.Signal\",\"uuid\":\"\"},{\"content\":{\"blockPath\":[],\"dimensions\":[1],\"domain\":\"\",\"lineColor\":\"#139fff\",\"plots\":[1],\"port\":2,\"sid\":[\"\"],\"signalID\":1091,\"signalName\":\"Demux2:2\"},\"type\":\"RecordBlkView.Signal\",\"uuid\":\"\"}]},\"type\":\"RecordBlkView.InputSignals\",\"uuid\":\"\"}],\"packageUris\":[\"http:\\/\\/schema.mathworks.com\\/mf0\\/streamout_blocks\\/R2020a\"],\"version\":\"1.0\"}"  VisualizationBindings="{\"xyplotplugin\":{\"info\":[{\"series\":[{\"bindingParametersList\":[{\"parameter\":\"X-Axis\",\"signalID\":1087,\"signalName\":\"Demux2:1\"},{\"parameter\":\"Y-Axis\",\"signalID\":1091,\"signalName\":\"Demux2:2\"}],\"seriesID\":46599}],\"subplotID\":1}]}}"  CompatibilityTag=XY
  a : Outport
  eabs : Outport  Port=2
  i : Outport  Port=3
  Raan : Outport  Port=4
  argp : Outport  Port=5
  nu : Outport  Port=6
  E : Outport  Port=7
  M : Outport  Port=8
  e : Outport  Port=9
  h : Outport  Port=10
  nu igen : Outport  Port=11
  s : Outport  Port=12
  wires:
  Subsystem5/1(nu) -> nu/1
  Subsystem1/3(Raan) -> Sum/2, 0 to 2*pi3/1(Raan), Raan/1
  Subsystem1/1(N) -> Subsystem4/3(N)  "N"
  Subsystem6/1(a) -> a/1
  Subsystem1/2(N_abs) -> Subsystem4/4(Nabs)  "Nabs"
  Subsystem3/1(e_vec) -> Selector1/1, e/1, Subsystem4/1(e), Subsystem5/2(e)  "e"
  Subsystem4/1(argp) -> Sum/1, argp/1
  Norm1/1(Out1) -> Subsystem6/2(vabs), Subsystem3/4(vabs)  "vabs"
  Subsystem2/1(i) -> i/1
  Cross Product/1 -> Subsystem1/1(h), Subsystem2/1(h), h/1  "h"
  v/1 -> Cross Product/2, Subsystem3/3(v), Subsystem/3(v), Norm1/1(In1)
  Subsystem3/2(e_abs) -> eabs/1, Subsystem5/3(eabs), Subsystem4/2(eabs)  "eabs"
  Norm2/1(Out1) -> Subsystem/2(rabs), Subsystem3/2(rabs), Subsystem6/1(rabs), Subsystem5/5(rabs)  "rabs"
  Subsystem5/2(M) -> M/1
  Subsystem5/4(nu igen) -> nu igen/1
  Subsystem5/3(E) -> E/1
  r/1 -> Selector/1, Subsystem/1(r), Norm2/1(In1), Cross Product/1, Subsystem5/4(r), Subsystem3/1(r)
  Subsystem/1(vr) -> Subsystem5/1(vr)
  Subsystem/2(vp) -> Terminator/1
  Trigonometric Function/1 -> 0 to 2*pi/1(In)  "truelong"
  Selector/1 -> Demux/1
  0 to 2*pi/1(Out) -> s/1  "s"
  Demux/1 -> Trigonometric Function/1
  Demux/2 -> Trigonometric Function/2
  Selector1/1 -> Demux1/1
  Trigonometric Function1/1 -> 0 to 2*pi1/1(In)  "truelong"
  Demux1/2 -> Trigonometric Function1/2
  0 to 2*pi1/1(Out) -> Gain/1  "truelong"
  Demux1/1 -> Trigonometric Function1/1
  Sum/1 -> 0 to 2*pi2/1(In)
  0 to 2*pi2/1(Out) -> Gain1/1  "truelong"
  Gain/1 -> Scope/1
  Gain1/1 -> Scope/2
  0 to 2*pi3/1(Out) -> Gain2/1  "truelong"
  Gain2/1 -> Scope/3
  Demux2/2 -> XY Graph/2
  Demux2/1 -> XY Graph/1
  Subsystem2/2(i_vec) -> Demux2/1

== system GEO_insertion/Subsystem1/Switch Case Action Subsystem/go to D = 0 ==
  D : Inport
  Constant : Constant  Value=A
  Constant1 : Constant  Value=psi_rads
  Constant2 : Constant  Value=-3*361
  Constant3 : Constant  Value=thrust_acc
  Divide : Product  Inputs=***/
  Divide1 : Product  Inputs=*/
  Divide2 : Product  Inputs=**
  Gain : Gain  Gain=1/(60*60*24)
  Gain1 : Gain  Gain=-1
  Gain2 : Gain  Gain=1/2
  dV (m/s) : Outport
  thrust_time (s) : Outport  Port=2
  dlambda_start (deg) : Outport  Port=3
  wires:
  D/1 -> Gain1/1
  Constant/1 -> Divide/2
  Constant1/1 -> Divide/3
  Constant2/1 -> Divide/4
  Divide/1 -> Divide1/1, dV (m/s)/1
  Constant3/1 -> Divide1/2
  Divide1/1 -> Gain2/1, thrust_time (s)/1
  Divide2/1 -> dlambda_start (deg)/1
  Gain1/1 -> Gain/1, Divide/1
  Gain/1 -> Divide2/1
  Gain2/1 -> Divide2/2

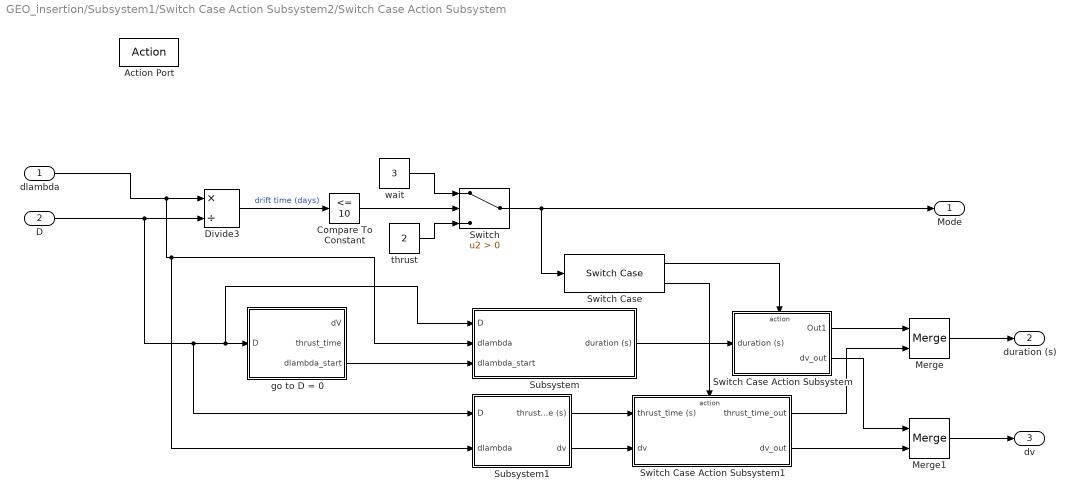
== system GEO_insertion/Subsystem1/Switch Case Action Subsystem2/Switch Case Action Subsystem ==
  dlambda : Inport
  D : Inport  Port=2
  Action Port : ActionPort  ActionPortLabel=case [ 1 ]:
  Compare To Constant : simulink/Logic and Bit Operations/Compare To Constant  relop=<=  const=10  OutDataTypeStr=boolean
  Divide3 : Product  Inputs=*/
  Merge : Merge
  Merge1 : Merge
  Subsystem : Subsystem
  Subsystem1 : Subsystem
  Switch : Switch  Criteria=u2 > Threshold  SaturateOnIntegerOverflow=off  InputSameDT=off
  Switch Case : SwitchCase  CaseConditions={3, 2}  ShowDefaultCase=off
  Switch Case Action Subsystem : Subsystem  TreatAsAtomicUnit=on
  Switch Case Action Subsystem1 : Subsystem  TreatAsAtomicUnit=on
  go to D = 0 : Subsystem
  thrust : Constant  Value=2
  wait : Constant  Value=3
  Mode : Outport
  duration (s) : Outport  Port=2
  dv : Outport  Port=3
  wires:
  Divide3/1 -> Compare To Constant/1  "drift time (days)"
  Compare To Constant/1 -> Switch/2
  dlambda/1 -> Subsystem1/2(dlambda), Subsystem/2(dlambda), Divide3/1
  D/1 -> Subsystem1/1(D), go to D = 0/1(D), Subsystem/1(D), Divide3/2
  wait/1 -> Switch/1
  Switch/1 -> Mode/1, Switch Case/1
  thrust/1 -> Switch/3
  Switch Case/1 -> Switch Case Action Subsystem/Action
  Switch Case Action Subsystem/1(Out1) -> Merge/1
  Merge/1 -> duration (s)/1
  Switch Case/2 -> Switch Case Action Subsystem1/Action
  Switch Case Action Subsystem1/1(thrust_time_out) -> Merge/2
  go to D = 0/3(dlambda_start) -> Subsystem/3(dlambda_start)
  Subsystem/1(duration (s)) -> Switch Case Action Subsystem/1(duration (s))
  Subsystem1/1(thrust_time (s)) -> Switch Case Action Subsystem1/1(thrust_time (s))
  Subsystem1/2(dv) -> Switch Case Action Subsystem1/2(dv)
  Switch Case Action Subsystem1/2(dv_out) -> Merge1/2
  Switch Case Action Subsystem/2(dv_out) -> Merge1/1
  Merge1/1 -> dv/1

== system GEO_insertion/Subsystem1/Switch Case Action Subsystem2/Switch Case Action Subsystem1 ==
  dlambda : Inport
  D : Inport  Port=2
  Action Port : ActionPort  ActionPortLabel=case [ 0 ]:
  Subsystem1 : Subsystem
  Thrust : Constant  Value=2
  Mode : Outport
  duration (s) : Outport  Port=2
  dv : Outport  Port=3
  wires:
  dlambda/1 -> Subsystem1/2(dlambda)
  D/1 -> Subsystem1/1(D)
  Subsystem1/1(thrust_time (s)) -> duration (s)/1
  Thrust/1 -> Mode/1
  Subsystem1/2(dv) -> dv/1

== system GEO_insertion/Subsystem/Subsystem2/Subsystem1/0 to 2*pi ==
  In : Inport
  Constant3 : Constant  Value=2*pi
  Math Function : Math  Operator=mod
  lambda : Outport
  wires:
  In/1 -> Math Function/1
  Math Function/1 -> lambda/1
  Constant3/1 -> Math Function/2

== system GEO_insertion/Subsystem/Subsystem2/Subsystem1/0 to 2*pi4 ==
  In : Inport
  Constant3 : Constant  Value=2*pi
  Math Function : Math  Operator=mod
  Out : Outport
  wires:
  In/1 -> Math Function/1
  Math Function/1 -> Out/1
  Constant3/1 -> Math Function/2

== system GEO_insertion/Subsystem/Subsystem2/Subsystem1/0 to 2*pi6 ==
  In : Inport
  Constant3 : Constant  Value=2*pi
  Math Function : Math  Operator=mod
  Out : Outport
  wires:
  In/1 -> Math Function/1
  Math Function/1 -> Out/1
  Constant3/1 -> Math Function/2

== system GEO_insertion/Subsystem/Subsystem2/Subsystem1/Norm3 ==
  In1 : Inport
  Dot Product : DotProduct  OutDataTypeStr=Inherit: Inherit via internal rule
  Sqrt : Sqrt
  Out1 : Outport
  wires:
  In1/1 -> Dot Product/1, Dot Product/2
  Sqrt/1 -> Out1/1
  Dot Product/1 -> Sqrt/1

== system GEO_insertion/Subsystem/Subsystem2/Subsystem1/Subsystem2 ==
  a : Inport
  Constant1 : Constant  Value=ext_ENV_muEarth
  Constant2 : Constant  Value=3
  Constant4 : Constant
  Divide : Product  Inputs=*/
  Gain1 : Gain  Gain=2*pi
  Gain4 : Gain  Gain=86164/2/pi
  Math Function : Math  Operator=pow
  Math Function1 : Math  Operator=reciprocal
  Sqrt : Sqrt
  Subtract : Sum  Inputs=+-
  lambdadot : Outport
  wires:
  Subtract/1 -> Gain1/1  "lambdadot"
  Constant4/1 -> Subtract/2
  Constant2/1 -> Math Function/2
  Sqrt/1 -> Math Function1/1
  Math Function/1 -> Divide/1
  Constant1/1 -> Divide/2
  a/1 -> Math Function/1
  Divide/1 -> Sqrt/1
  Math Function1/1 -> Gain4/1
  Gain4/1 -> Subtract/1
  Gain1/1 -> lambdadot/1

== system GEO_insertion/Subsystem/Subsystem2/Subsystem7/0 to 2*pi ==
  In : Inport
  Constant3 : Constant  Value=2*pi
  Math Function : Math  Operator=mod
  Out : Outport
  wires:
  In/1 -> Math Function/1
  Math Function/1 -> Out/1
  Constant3/1 -> Math Function/2

== system GEO_insertion/Subsystem/Subsystem2/Subsystem7/0 to 2*pi1 ==
  In : Inport
  Constant3 : Constant  Value=2*pi
  Math Function : Math  Operator=mod
  Out : Outport
  wires:
  In/1 -> Math Function/1
  Math Function/1 -> Out/1
  Constant3/1 -> Math Function/2

== system GEO_insertion/Subsystem/Subsystem2/Subsystem7/0 to 2*pi2 ==
  In : Inport
  Constant3 : Constant  Value=2*pi
  Math Function : Math  Operator=mod
  Out : Outport
  wires:
  In/1 -> Math Function/1
  Math Function/1 -> Out/1
  Constant3/1 -> Math Function/2

== system GEO_insertion/Subsystem/Subsystem2/Subsystem7/0 to 2*pi3 ==
  Raan : Inport
  Constant3 : Constant  Value=2*pi
  Math Function : Math  Operator=mod
  Out : Outport
  wires:
  Raan/1 -> Math Function/1
  Math Function/1 -> Out/1
  Constant3/1 -> Math Function/2

== system GEO_insertion/Subsystem/Subsystem2/Subsystem7/Norm1 ==
  In1 : Inport
  Dot Product : DotProduct  OutDataTypeStr=Inherit: Inherit via internal rule
  Sqrt : Sqrt
  Out1 : Outport
  wires:
  In1/1 -> Dot Product/1, Dot Product/2
  Sqrt/1 -> Out1/1
  Dot Product/1 -> Sqrt/1

== system GEO_insertion/Subsystem/Subsystem2/Subsystem7/Norm2 ==
  In1 : Inport
  Dot Product : DotProduct  OutDataTypeStr=Inherit: Inherit via internal rule
  Sqrt : Sqrt
  Out1 : Outport
  wires:
  In1/1 -> Dot Product/1, Dot Product/2
  Sqrt/1 -> Out1/1
  Dot Product/1 -> Sqrt/1

== system GEO_insertion/Subsystem/Subsystem2/Subsystem7/Subsystem ==
  r : Inport
  rabs : Inport  Port=2
  v : Inport  Port=3
  Divide : Product  Inputs=*/
  Dot Product : DotProduct  OutDataTypeStr=Inherit: Inherit via internal rule
  Dot Product1 : DotProduct  OutDataTypeStr=Inherit: Inherit via internal rule
  Math Function : Math  Operator=square
  Sqrt : Sqrt
  Subtract1 : Sum  Inputs=+-
  vr : Outport
  vp : Outport  Port=2
  wires:
  Sqrt/1 -> vp/1  "vp"
  rabs/1 -> Divide/2
  Subtract1/1 -> Sqrt/1
  r/1 -> Divide/1
  Dot Product1/1 -> Subtract1/1  "vr"
  Divide/1 -> Dot Product/1
  Math Function/1 -> Subtract1/2
  v/1 -> Dot Product/2, Dot Product1/1, Dot Product1/2
  Dot Product/1 -> vr/1, Math Function/1  "vr"

== system GEO_insertion/Subsystem/Subsystem2/Subsystem7/Subsystem1 ==
  h : Inport
  Constant : Constant  Value=0
  Divide2 : Product  Inputs=*/
  Mux : Mux  Inputs=3
  Norm4 : Subsystem  Tag=||u||
      mask Display: disp('||u||')
  Selector1 : Selector  InputPortWidth=3  IndexOptions=Index vector (dialog)  Indices=[2]  OutputSizes=1
  Selector2 : Selector  InputPortWidth=3  IndexOptions=Index vector (dialog)  Indices=[1]  OutputSizes=1
  Selector3 : Selector  InputPortWidth=3  IndexOptions=Index vector (dialog)  Indices=[1]  OutputSizes=1
  Trigonometric Function1 : Trigonometry  Operator=acos
  Unary Minus : UnaryMinus
  N : Outport
  N_abs : Outport  Port=2
  Raan : Outport  Port=3
  wires:
  Trigonometric Function1/1 -> Raan/1  "Raan"
  Unary Minus/1 -> Mux/1
  Selector1/1 -> Unary Minus/1
  Divide2/1 -> Trigonometric Function1/1
  Norm4/1(Out1) -> Divide2/2, N_abs/1  "N_abs"
  Constant/1 -> Mux/3
  Selector3/1 -> Divide2/1
  Selector2/1 -> Mux/2
  h/1 -> Selector2/1, Selector1/1
  Mux/1 -> N/1, Selector3/1, Norm4/1(In1)  "N"

== system GEO_insertion/Subsystem/Subsystem2/Subsystem7/Subsystem2 ==
  h : Inport
  Divide1 : Product  Inputs=*/
  Divide2 : Product  Inputs=*/
  Divide3 : Product  Inputs=**
  Norm1 : Subsystem  Tag=||u||
      mask Display: disp('||u||')
  Norm3 : Subsystem  Tag=||u||
      mask Display: disp('||u||')
  Selector : Selector  InputPortWidth=3  IndexOptions=Index vector (dialog)  Indices=[3]  OutputSizes=1
  Selector1 : Selector  InputPortWidth=3  IndexOptions=Index vector (dialog)  Indices=[1 2]  OutputSizes=1
  Trigonometric Function : Trigonometry  Operator=acos
  i : Outport
  i_vec : Outport  Port=2
  wires:
  Trigonometric Function/1 -> Divide3/1, i/1  "i"
  Selector/1 -> Divide1/1
  h/1 -> Selector1/1, Norm3/1(In1), Selector/1
  Norm3/1(Out1) -> Divide1/2
  Divide1/1 -> Trigonometric Function/1
  Selector1/1 -> Norm1/1(In1), Divide2/1
  Norm1/1(Out1) -> Divide2/2
  Divide2/1 -> Divide3/2
  Divide3/1 -> i_vec/1

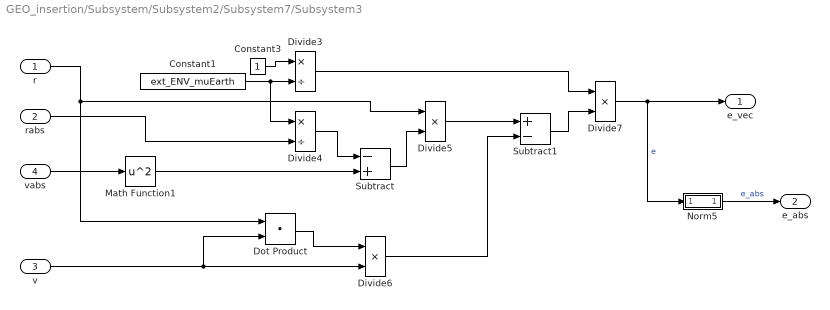
== system GEO_insertion/Subsystem/Subsystem2/Subsystem7/Subsystem3 ==
  r : Inport
  rabs : Inport  Port=2
  v : Inport  Port=3
  vabs : Inport  Port=4
  Constant1 : Constant  Value=ext_ENV_muEarth
  Constant3 : Constant
  Divide3 : Product  Inputs=*/
  Divide4 : Product  Inputs=*/
  Divide5 : Product  Inputs=**
  Divide6 : Product  Inputs=**
  Divide7 : Product  Inputs=**
  Dot Product : DotProduct  OutDataTypeStr=Inherit: Inherit via internal rule
  Math Function1 : Math  Operator=square
  Norm5 : Subsystem  Tag=||u||
      mask Display: disp('||u||')
  Subtract : Sum  Inputs=-+
  Subtract1 : Sum  Inputs=+-
  e_vec : Outport
  e_abs : Outport  Port=2
  wires:
  rabs/1 -> Divide4/2
  r/1 -> Dot Product/1, Divide5/1
  Subtract1/1 -> Divide7/2
  Norm5/1(Out1) -> e_abs/1  "e_abs"
  Divide7/1 -> Norm5/1(In1), e_vec/1  "e"
  Constant3/1 -> Divide3/1
  vabs/1 -> Math Function1/1
  Constant1/1 -> Divide4/1, Divide3/2
  Subtract/1 -> Divide5/2
  Divide5/1 -> Subtract1/1
  Divide4/1 -> Subtract/1
  v/1 -> Dot Product/2, Divide6/2
  Divide6/1 -> Subtract1/2
  Dot Product/1 -> Divide6/1
  Math Function1/1 -> Subtract/2
  Divide3/1 -> Divide7/1

== system GEO_insertion/Subsystem/Subsystem2/Subsystem7/Subsystem4 ==
  e : Inport
  eabs : Inport  Port=2
  N : Inport  Port=3
  Nabs : Inport  Port=4
  Divide8 : Product  Inputs=*/
  Divide9 : Product  Inputs=**
  Dot Product1 : DotProduct  OutDataTypeStr=Inherit: Inherit via internal rule
  Trigonometric Function2 : Trigonometry  Operator=acos
  argp : Outport
  wires:
  Nabs/1 -> Divide9/2
  N/1 -> Dot Product1/2
  Divide9/1 -> Divide8/2  "e"
  Trigonometric Function2/1 -> argp/1  "argp"
  Dot Product1/1 -> Divide8/1
  e/1 -> Dot Product1/1
  eabs/1 -> Divide9/1
  Divide8/1 -> Trigonometric Function2/1

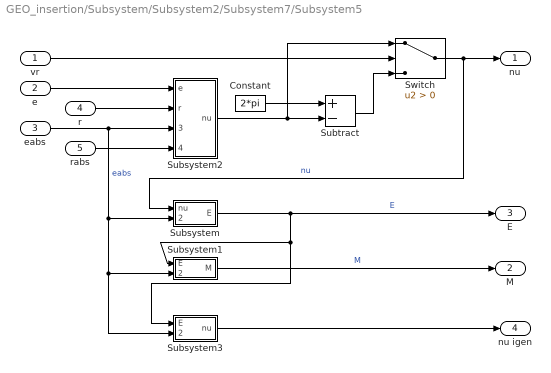
== system GEO_insertion/Subsystem/Subsystem2/Subsystem7/Subsystem5 ==
  vr : Inport
  e : Inport  Port=2
  eabs : Inport  Port=3
  r : Inport  Port=4
  rabs : Inport  Port=5
  Constant : Constant  Value=2*pi
  Subsystem : Subsystem
  Subsystem1 : Subsystem
  Subsystem2 : Subsystem
  Subsystem3 : Subsystem
  Subtract : Sum  Inputs=+-
  Switch : Switch  Criteria=u2 > Threshold  SaturateOnIntegerOverflow=off  InputSameDT=off
  nu : Outport
  M : Outport  Port=2
  E : Outport  Port=3
  nu igen : Outport  Port=4
  wires:
  eabs/1 -> Subsystem1/2(eabs), Subsystem3/2(eabs), Subsystem/2(eabs), Subsystem2/3(eabs)  "eabs"
  Subsystem/1(E) -> Subsystem1/1(E), Subsystem3/1(E), E/1  "E"
  Subsystem2/1(nu) -> Switch/1, Subtract/2
  e/1 -> Subsystem2/1(e)
  r/1 -> Subsystem2/2(r)
  rabs/1 -> Subsystem2/4(rabs)
  Subsystem3/1(nu) -> nu igen/1
  vr/1 -> Switch/2
  Switch/1 -> nu/1, Subsystem/1(nu)  "nu"
  Constant/1 -> Subtract/1
  Subtract/1 -> Switch/3
  Subsystem1/1(M) -> M/1  "M"

== system GEO_insertion/Subsystem/Subsystem2/Subsystem7/Subsystem6 ==
  rabs : Inport
  vabs : Inport  Port=2
  Constant3 : Constant
  Constant4 : Constant  Value=2
  Constant5 : Constant  Value=ext_ENV_muEarth
  Divide1 : Product  Inputs=*/
  Divide3 : Product  Inputs=*/
  Divide4 : Product  Inputs=*/
  Math Function1 : Math  Operator=square
  Subtract : Sum  Inputs=+-
  a : Outport
  wires:
  Divide3/1 -> a/1  "a"
  vabs/1 -> Math Function1/1
  Divide4/1 -> Subtract/1
  Math Function1/1 -> Divide1/1
  Constant4/1 -> Divide4/1
  rabs/1 -> Divide4/2
  Divide1/1 -> Subtract/2
  Subtract/1 -> Divide3/2
  Constant3/1 -> Divide3/1
  Constant5/1 -> Divide1/2

== system GEO_insertion/Subsystem1/Switch Case Action Subsystem2/Switch Case Action Subsystem/Subsystem ==
  D : Inport
  dlambda : Inport  Port=2
  dlambda_start : Inport  Port=3
  Divide : Product  Inputs=*/
  Subtract : Sum  Inputs=+-
  days 2 sec : Gain  Gain=60*60*24
  duration (s) : Outport
  wires:
  dlambda/1 -> Subtract/1
  dlambda_start/1 -> Subtract/2
  Subtract/1 -> Divide/1
  D/1 -> Divide/2
  Divide/1 -> days 2 sec/1
  days 2 sec/1 -> duration (s)/1

== system GEO_insertion/Subsystem1/Switch Case Action Subsystem2/Switch Case Action Subsystem/Subsystem1 ==
  D : Inport
  dlambda : Inport  Port=2
  Constant : Constant  Value=10
  Divide : Product  Inputs=*/
  Subtract : Sum  Inputs=+-
  go to D = 0 : Subsystem
  thrust_time (s) : Outport
  dv : Outport  Port=2
  wires:
  dlambda/1 -> Divide/1
  Constant/1 -> Divide/2
  Divide/1 -> Subtract/1
  D/1 -> Subtract/2
  Subtract/1 -> go to D = 0/1(D)
  go to D = 0/2(thrust_time (s)) -> thrust_time (s)/1
  go to D = 0/1(dV (m/s)) -> dv/1

== system GEO_insertion/Subsystem1/Switch Case Action Subsystem2/Switch Case Action Subsystem/Switch Case Action Subsystem ==
  duration (s) : Inport
  Action Port : ActionPort  ActionPortLabel=case [ 3 ]:
  Constant : Constant  Value=0
  Out1 : Outport
  dv_out : Outport  Port=2
  wires:
  duration (s)/1 -> Out1/1
  Constant/1 -> dv_out/1

== system GEO_insertion/Subsystem1/Switch Case Action Subsystem2/Switch Case Action Subsystem/Switch Case Action Subsystem1 ==
  thrust_time (s) : Inport
  dv : Inport  Port=2
  Action Port : ActionPort  ActionPortLabel=case [ 2 ]:
  thrust_time_out : Outport
  dv_out : Outport  Port=2
  wires:
  thrust_time (s)/1 -> thrust_time_out/1
  dv/1 -> dv_out/1

== system GEO_insertion/Subsystem1/Switch Case Action Subsystem2/Switch Case Action Subsystem/go to D = 0 ==
  D : Inport
  Constant : Constant  Value=A
  Constant1 : Constant  Value=psi_rads
  Constant2 : Constant  Value=-3*361
  Constant3 : Constant  Value=thrust_acc
  Divide : Product  Inputs=***/
  Divide1 : Product  Inputs=*/
  Divide2 : Product  Inputs=*/
  Gain : Gain  Gain=1/2
  dV : Outport
  thrust_time : Outport  Port=2
  dlambda_start : Outport  Port=3
  wires:
  D/1 -> Divide2/1, Divide/1
  Constant/1 -> Divide/2
  Constant1/1 -> Divide/3
  Constant2/1 -> Divide/4
  Divide/1 -> Divide1/1, dV/1
  Constant3/1 -> Divide1/2
  Divide1/1 -> Gain/1, thrust_time/1
  Gain/1 -> Divide2/2
  Divide2/1 -> dlambda_start/1

== system GEO_insertion/Subsystem1/Switch Case Action Subsystem2/Switch Case Action Subsystem1/Subsystem1 ==
  D : Inport
  dlambda : Inport  Port=2
  Constant : Constant  Value=10
  Divide : Product  Inputs=*/
  Subtract : Sum  Inputs=+-
  go to D = 0 : Subsystem
  thrust_time (s) : Outport
  dv : Outport  Port=2
  wires:
  dlambda/1 -> Divide/1
  Constant/1 -> Divide/2
  Divide/1 -> Subtract/1
  D/1 -> Subtract/2
  Subtract/1 -> go to D = 0/1(D)
  go to D = 0/2(thrust_time (s)) -> thrust_time (s)/1
  go to D = 0/1(dV (m/s)) -> dv/1

== system GEO_insertion/Subsystem/Subsystem2/Subsystem7/Subsystem1/Norm4 ==
  In1 : Inport
  Dot Product : DotProduct  OutDataTypeStr=Inherit: Inherit via internal rule
  Sqrt : Sqrt
  Out1 : Outport
  wires:
  In1/1 -> Dot Product/1, Dot Product/2
  Sqrt/1 -> Out1/1
  Dot Product/1 -> Sqrt/1

== system GEO_insertion/Subsystem/Subsystem2/Subsystem7/Subsystem2/Norm1 ==
  In1 : Inport
  Dot Product : DotProduct  OutDataTypeStr=Inherit: Inherit via internal rule
  Sqrt : Sqrt
  Out1 : Outport
  wires:
  In1/1 -> Dot Product/1, Dot Product/2
  Sqrt/1 -> Out1/1
  Dot Product/1 -> Sqrt/1

== system GEO_insertion/Subsystem/Subsystem2/Subsystem7/Subsystem2/Norm3 ==
  In1 : Inport
  Dot Product : DotProduct  OutDataTypeStr=Inherit: Inherit via internal rule
  Sqrt : Sqrt
  Out1 : Outport
  wires:
  In1/1 -> Dot Product/1, Dot Product/2
  Sqrt/1 -> Out1/1
  Dot Product/1 -> Sqrt/1

== system GEO_insertion/Subsystem/Subsystem2/Subsystem7/Subsystem3/Norm5 ==
  In1 : Inport
  Dot Product : DotProduct  OutDataTypeStr=Inherit: Inherit via internal rule
  Sqrt : Sqrt
  Out1 : Outport
  wires:
  In1/1 -> Dot Product/1, Dot Product/2
  Sqrt/1 -> Out1/1
  Dot Product/1 -> Sqrt/1
